simulink model "Tutorial28"  (R2020a)
settings: Solver=FixedStepDiscrete  StartTime=0  StopTime=1  FixedStep=0.1  RelTol=1e-3
libraries: dspsrcs4 x3
settings Model: Creator=ashok  LastModifiedBy=ashok

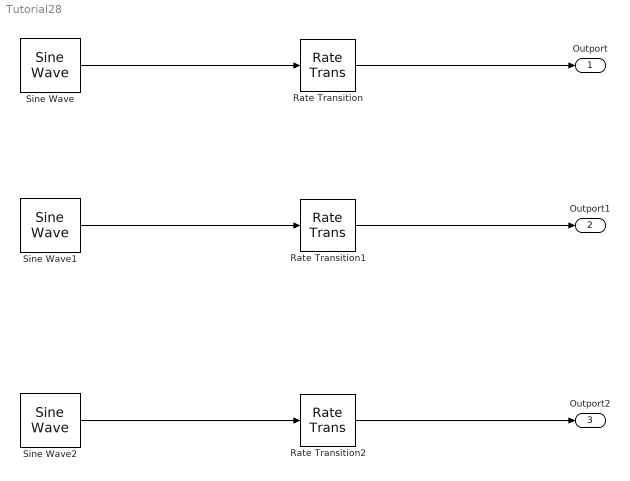
== system Tutorial28 ==
  Rate Transition : RateTransition
  Rate Transition1 : RateTransition
  Rate Transition2 : RateTransition
  Sine Wave : dspsrcs4/Sine Wave  Amplitude=4  Frequency=100  Phase=0  SampleMode=Discrete  OutComplex=Real  CompMethod=Trigonometric fcn  TableSize=Speed  SampleTime=0.1  SamplesPerFrame=1  ResetState=Restart at time zero  OutputFrames=off  dataType=double  wordLen=16  udDataType=sfix(16)  fracBitsMode=Best precision  numFracBits=15  OutDataTypeStr=double  LastOutDataTypeStr=double
  Sine Wave1 : dspsrcs4/Sine Wave  Amplitude=4  Frequency=100  Phase=0  SampleMode=Discrete  OutComplex=Real  CompMethod=Trigonometric fcn  TableSize=Speed  SampleTime=0.2  SamplesPerFrame=1  ResetState=Restart at time zero  OutputFrames=off  dataType=double  wordLen=16  udDataType=sfix(16)  fracBitsMode=Best precision  numFracBits=15  OutDataTypeStr=double  LastOutDataTypeStr=double
  Sine Wave2 : dspsrcs4/Sine Wave  Amplitude=4  Frequency=100  Phase=0  SampleMode=Discrete  OutComplex=Real  CompMethod=Trigonometric fcn  TableSize=Speed  SampleTime=0.3  SamplesPerFrame=1  ResetState=Restart at time zero  OutputFrames=off  dataType=double  wordLen=16  udDataType=sfix(16)  fracBitsMode=Best precision  numFracBits=15  OutDataTypeStr=double  LastOutDataTypeStr=double
  Outport : Outport  SampleTime=0.2
  Outport1 : Outport  Port=2  SampleTime=0.1
  Outport2 : Outport  Port=3  SampleTime=0.3
  wires:
  Sine Wave/1 -> Rate Transition/1
  Rate Transition/1 -> Outport/1
  Rate Transition1/1 -> Outport1/1
  Sine Wave1/1 -> Rate Transition1/1
  Sine Wave2/1 -> Rate Transition2/1
  Rate Transition2/1 -> Outport2/1
